simulink model "CAN_Tx"  (R2018b)
settings: Solver=FixedStepDiscrete  StartTime=0.0  StopTime=10.0  FixedStep=0.005  RelTol=1e-3
PostLoadFcn:
  | if any(exist('dsrtsu_mdlpostloadfcn', 'file') ~= 0), dsrtsu_mdlpostloadfcn('Execute', bdroot); end
values from neighbouring files (symbols this model uses):
  P_x165_On = 1.0    [CAN_Tx.sldd]
  P_x242_On = 1.0    [CAN_Tx.sldd]
  P_x246_On = 1.0    [CAN_Tx.sldd]
libraries: simulink x23, rtican x16
(part 2 of 4)

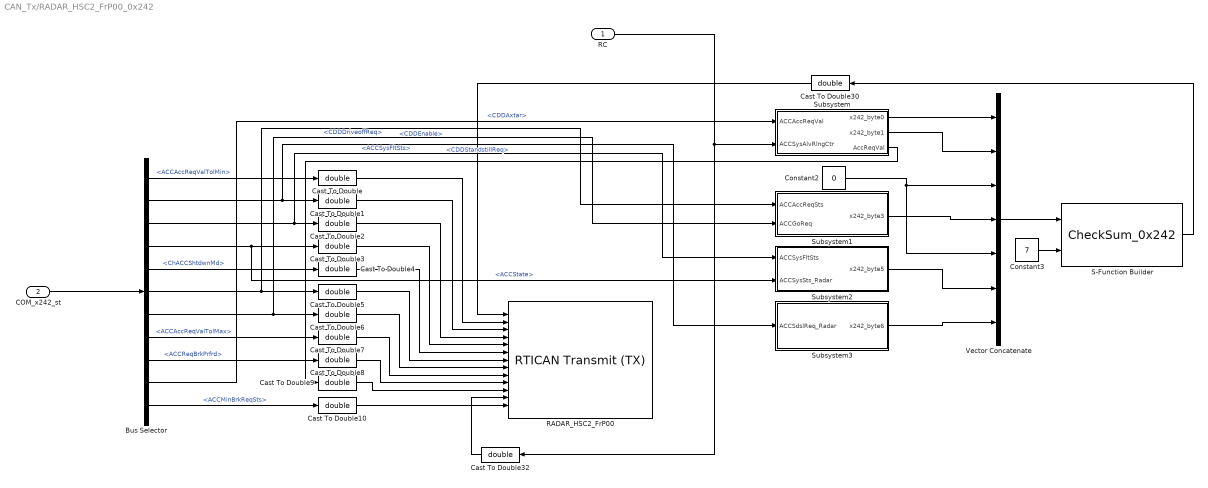
== system CAN_Tx/RADAR_HSC2_FrP00_0x242 ==
  RC : Inport
  COM_x242_st : Inport  Port=2
  Bus Selector : BusSelector  OutputSignals=ACCAccReqValTolMin,CDDStandstillReq,ACCSysFltSts,ACCState,ChACCShtdwnMd,CDDEnable,CDDDriveoffReq,ACCAccReqValTolMax,ACCReqBrkPrfrd,CDDAxtar,ACCMinBrkReqSts
  Cast To Double{,1..10,30,32} (13 alike) : DataTypeConversion  OutDataTypeStr=double
  Constant2 : Constant  Value=0  OutDataTypeStr=uint8
  Constant3 : Constant  Value=7  OutDataTypeStr=uint8
  RADAR_HSC2_FrP00 : rtican/RTICAN Transmit (TX)   Reserved1=[]  Reserved2=[]  Reserved3=[]  Reserved4=[]  SfcnMessage=[]  Msg_Struct=[]  BoardTypeNo=[]  BoardNo=[]  ChannelNo=[]  Parameters=[]  DialogFcn=[]  UnitName=[]  Revision=[]  UnitValues=[]  DSProperties=struct('RTI',struct('Version',uint32(5),'BlockType',struct('isSLSource',uint8(1),'isSLSink',uint8(1),'isHWSource',uint8(0),'isHWSink',uint8(0),'isSetup',uint8(0),'isInline',uint8(1),'isNonInline',uint8(0),'isInterrupt',uint8(0),'isChannelwise',uint8(0)),'IOBoardType','RTICAN','UnitType','MESSAGE','Identifier','TX','DialogType','MSVC','BlockSet','RTICAN','SlaveProcessor','CAN'))  RTIBlockInterface=struct('InputPortsWidth',int32([1 1 1 1 1 1 1 1 1 1 1 1 1]),'InputPortsActive',ones(1,13),'InputPortsName',{{'ACCSysChksm_SCSHSC2','ACCAccReqValTolMinHSC2','ACCSdslReq_RadarHSC2','ACCSysFltSts_SCSHSC2','ACCSysSts_RadarHSC2','ChACCShtdwnMdHSC2','ACCAccReqStsHSC2','ACCGoReqHSC2','ACCAccReqValTolMaxHSC2','ACCReqBrkPrfrdHSC2','ACCAccReqValHSC2','ACCSysAlvRlngCtr_SCSHSC2','ACCMinBrkReqStsHSC2'}},'InputPortsDataType',{{'SS_DOUBLE','SS_DOUBLE','SS_DOUBLE','SS_DOUBLE','SS_DOUBLE','SS_DOUBLE','SS_DOUBLE','SS_DOUBLE','SS_DOUBLE','SS_DOUBLE','SS_DOUBLE','SS_DOUBLE','SS_DOUBLE'}},'OutputPortsWidth',int32([1 1 1 1]),'OutputPortsActive',[1 1 1 1],'OutputPortsName',{{['TX status'],['TX time'],['TX delta time'],['TX delay time']}},'DialogFcn','rtican_message_interface_gui','BlockDisplay',{{'','center'}},'IconTransparency','on','InitLevel',3,'BlockName',struct('Token',{{'RADAR_HSC2_FrP00'}}),'SampleTime',{{-1}},'TriggerPort',{{'none'}},'EnablePort',{{'none'}})  RTIBlockParameters=struct('BoardTypeNo',{{1,'OFF',[]}},'BoardNo',{{1,'ON',[1 16]}},'ChannelNo',{{1,'ON',[1 2]}},'Parameters',{{struct('DataFileSupport',struct('DataFileSelectedMaster',1,'DataFileSelectedLocal',1,'DataFileName','c:\users\administrator.zx-201607042142\desktop\zone\2020_demo\ep21原车dbc\171114-lh1-ep21_ep2_fdr-_v07.dbc|','DataFileDate',['24-11月-2020 08:54:40'],'SelectedFile','..\..\dbc\ep21_dbc\171114-lh1-ep21_ep2_fdr-_v07_acc.dbc','InterfaceFcn','rtican_dbc_file_parser'),'Options',struct('StatusSelected',1,'TimeSelected',1,'DeltaTimeSelected',1,'DelayTimeSelected',1,'DelayTimeTXCommandSelected',0,'EncodeSetUnusedBitsToOne',0,'EnableMsgLoopback',0,'TriggerPort',struct('Selected',0,'TriggerType',0),'EnablePortSelected',0,'SignalOnPortnameSelected',1,'UserCoding',struct('Selected',0,'InterfaceFile','UserEncodingFile','FcnName','UserEncodeFcn','InportSelected',0,'InportWidth',1,'OutportSelected',0,'OutportWidth',1),'TerminationMsg',struct('Selected',0,'Byte0_7','0'),'InitialMsg',struct('Selected',0,'Byte0_7','0')),'Message',struct('MsgOnBlocknameSelected',1,'MsgName','RADAR_HSC2_FrP00','MsgIdFormat',0,'MsgId',578,'MsgLength',8,'NumSignals',13,'SampleTime',-1,'StartTime',struct('Selected',0,'Value',3),'AutoRepeatTime',struct('Selected',0,'Value',0.1),'Timeout',struct('Selected',0,'Value',0.1),'DelayTime',struct('Selected',0,'Value',0.1),'Signal',struct('SgnName',{'ACCSysChksm_SCSHSC2','ACCAccReqValTolMinHSC2','ACCSdslReq_RadarHSC2','ACCSysFltSts_SCSHSC2','ACCSysSts_RadarHSC2','ChACCShtdwnMdHSC2','ACCAccReqStsHSC2','ACCGoReqHSC2','ACCAccReqValTolMaxHSC2','ACCReqBrkPrfrdHSC2','ACCAccReqValHSC2','ACCSysAlvRlngCtr_SCSHSC2','ACCMinBrkReqStsHSC2'},'SgnStartBit',{0,8,15,16,19,22,36,38,40,47,48,59,63},'SgnLength',{8,7,1,3,3,2,2,1,7,1,11,4,1},'ByteLayout',{2,2,2,2,2,2,2,2,2,2,2,2,2},'Factor',{1,0.025,1,1,1,1,1,1,0.025,1,0.005,1,1},'Offset',{0,0,0,0,0,0,0,0,0,0,-7.22,0,0},'SgnComment',{'','','','','','',['Adaptive Cruise Control Acceleration Request Status'],['Adaptive Cruise Control Go Request'],'','','','',''},'SgnUnit',{'','','','','','','','','','','','',''},'Min',{0,0,0,0,0,0,0,0,0,0,-7.22,0,0},'Max',{255,3.175,1,7,7,3,3,1,3.175,1,3.015,15,1},'SgnType',{0,0,0,0,0,0,0,0,0,0,0,0,0},'SLDataType',{'SS_DOUBLE','SS_DOUBLE','SS_DOUBLE','SS_DOUBLE','SS_DOUBLE','SS_DOUBLE','SS_DOUBLE','SS_DOUBLE','SS_DOUBLE','SS_DOUBLE','SS_DOUBLE','SS_DOUBLE','SS_DOUBLE'},'DataType',{0,0,0,0,0,0,0,0,0,0,0,0,0},'ModeValue',{-1,-1,-1,-1,-1,-1,-1,-1,-1,-1,-1,-1,-1}),'MsgIdNumFormat',0,'MsgComment',{{''}}),'Version',1.2,'general',struct('isFromLib',0)),'OFF',[]}},'GroupId',{{struct('Group',{{'RTICAN'}},'No',1,'Behavior',{{'NAMECHANGE'}},'BlockType',{{'SINK'}},'NameChangeFlag',0),'OFF',[]}},'SFcnRTICANMessage',{{struct('MsgType','TX','SFcnPortType','Scalar','MsgName','RADAR_HSC2_FrP00','MsgIdFormat','STD','MsgId',578,'MsgLength',8,'NumSignals',13,'SampleTime',-1,'StartTime',struct('Selected','no','Value',3),'AutoRepeatTime',struct('Selected','no','Value',0.1),'Timeout',struct('Selected','no','Value',0.1),'Signal',struct('SgnName',{'ACCSysChksm_SCSHSC2','ACCAccReqValTolMinHSC2','ACCSdslReq_RadarHSC2','ACCSysFltSts_SCSHSC2','ACCSysSts_RadarHSC2','ChACCShtdwnMdHSC2','ACCAccReqStsHSC2','ACCGoReqHSC2','ACCAccReqValTolMaxHSC2','ACCReqBrkPrfrdHSC2','ACCAccReqValHSC2','ACCSysAlvRlngCtr_SCSHSC2','ACCMinBrkReqStsHSC2'},'SgnStartBit',{0,8,15,16,19,22,36,38,40,47,48,59,63},'SgnLength',{8,7,1,3,3,2,2,1,7,1,11,4,1},'ByteLayout',{['motorola back.'],['motorola back.'],['motorola back.'],['motorola back.'],['motorola back.'],['motorola back.'],['motorola back.'],['motorola back.'],['motorola back.'],['motorola back.'],['motorola back.'],['motorola back.'],['motorola back.']},'Factor',{1,0.025,1,1,1,1,1,1,0.025,1,0.005,1,1},'Offset',{0,0,0,0,0,0,0,0,0,0,-7.22,0,0},'SgnType',{'standard','standard','standard','standard','standard','standard','standard','standard','standard','standard','standard','standard','standard'},'SLDataType',{'SS_DOUBLE','SS_DOUBLE','SS_DOUBLE','SS_DOUBLE','SS_DOUBLE','SS_DOUBLE','SS_DOUBLE','SS_DOUBLE','SS_DOUBLE','SS_DOUBLE','SS_DOUBLE','SS_DOUBLE','SS_DOUBLE'},'DataType',{['unsigned int'],['unsigned int'],['unsigned int'],['unsigned int'],['unsigned int'],['unsigned int'],['unsigned int'],['unsigned int'],['unsigned int'],['unsigned int'],['unsigned int'],['unsigned int'],['unsigned int']},'ModeValue',{-1,-1,-1,-1,-1,-1,-1,-1,-1,-1,-1,-1,-1}),'StatusSelected','yes','TimeSelected','yes','DeltaTimeSelected','yes','DelayTimeSelected','yes','DelayTimeTXCommandSelected','no','EncodeSetUnusedBitsToOne','no','EnableMsgLoopback','no','TriggerPort',struct('Selected','no','TriggerType',0),'EnablePortSelected','no','UserCoding',struct('Selected','no','InterfaceFile','UserEncodingFile','FcnName','UserEncodeFcn','InportSelected','no','InportWidth',1,'OutportSelected','no','OutportWidth',1),'TerminationMsg',struct('Selected','no','Byte0','0x00','Byte1','0x00','Byte2','0x00','Byte3','0x00','Byte4','0x00','Byte5','0x00','Byte6','0x00','Byte7','0x00'),'InitialMsg',struct('Selected','no','Byte0','0x00','Byte1','0x00','Byte2','0x00','Byte3','0x00','Byte4','0x00','Byte5','0x00','Byte6','0x00','Byte7','0x00'),'BoardType','DS1','BoardNo',1,'ControllerNo',1),'OFF',[]}},'TLCFileName',{{'rtican_tx_message','OFF',[]}})  RTISFcnParameters=struct('SFcnRTICANMessage','struct','TLCFileName','char')  RTIBlockParaDefault=struct('BoardTypeNo',4302,'BoardNo',1,'ChannelNo',1,'Parameters',struct('DataFileSupport',struct('DataFileSelectedMaster',0,'DataFileSelectedLocal',0,'DataFileName','','DataFileDate','','SelectedFile',['<no file selected>']),'Options',struct('StatusSelected',1,'TimeSelected',1,'DeltaTimeSelected',1,'DelayTimeSelected',1,'DelayTimeTXCommandSelected',0,'EncodeSetUnusedBitsToOne',0,'EnableMsgLoopback',0,'TriggerPort',struct('Selected',0,'TriggerType','rising'),'EnablePortSelected',0,'SignalOnPortnameSelected',1,'UserCoding',struct('Selected',0,'InterfaceFile','UserEncodingFile','FcnName','UserEncodeFcn','InportSelected',0,'InportWidth',1,'OutportSelected',0,'OutportWidth',1),'TerminationMsg',struct('Selected',0,'Byte0_7','0'),'InitialMsg',struct('Selected',0,'Byte0_7','0')),'Message',struct('MsgOnBlocknameSelected',0,'MsgName',['TX Message'],'MsgIdFormat',0,'MsgId',100,'MsgLength',8,'NumSignals',1,'SampleTime',-1,'StartTime',struct('Selected',0,'Value',0),'AutoRepeatTime',struct('Selected',0,'Value',0.1),'Timeout',struct('Selected',0,'Value',0.1),'DelayTime',struct('Selected',0,'Value',0.1),'Signal',struct('SgnName',['TX signal'],'SgnStartBit',0,'SgnLength',8,'SgnType',0,'ModeValue',-1,'DataType',0,'SLDataType','SS_DOUBLE','ByteLayout',0,'Factor',1,'Offset',0,'Min',0,'Max',255,'SgnComment',{{}},'SgnUnit',''),'MsgIdNumFormat',0,'MsgComment',{{''}}),'Version',1.2,'general',struct('isFromLib',1)),'GroupId',struct('Group',{{'RTICAN'}},'No',1,'Behavior',{{'NAMECHANGE'}},'BlockType',{{'SINK'}},'NameChangeFlag',0),'SFcnRTICANMessage',struct('MsgType','TX','MsgName',['TX Message'],'MsgIdFormat','STD','MsgId',100,'MsgLength',2,'NumSignals',1,'SampleTime',-1,'StartTime',struct('Selected','no','Value',0),'AutoRepeatTime',struct('Selected','no','Value',0.1),'Timeout',struct('Selected','no','Value',0.1),'DelayTime',struct('Selected','no','Value',0.1),'Signal',struct('SgnName',['TX signal'],'SgnStartBit',0,'SgnLength',8,'SgnType','standard','ModeValue',-1,'DataType',['unsigned int'],'ByteLayout',['little endian'],'SLDataType','SS_DOUBLE','Factor',1,'Offset',0),'StatusSelected','yes','TimeSelected','yes','DeltaTimeSelected','yes','DelayTimeSelected','yes','EnablePortSelected','no','EnableMsgLoopback','no','DelayTimeTXCommandSelected','no','EncodeSetUnusedBitsToOne','no','UserCoding',struct('Selected','no','InterfaceFile','UserDecodingFile','FcnName','UserDecodeFcn','InportSelected','no','InportWidth',1,'OutportSelected','no','OutportWidth',1),'TerminationMsg',struct('Selected','no','Byte0','0x00','Byte1','0x00','Byte2','0x00','Byte3','0x00','Byte4','0x00','Byte5','0x00','Byte6','0x00','Byte7','0x00'),'InitialMsg',struct('Selected','no','Byte0','0x00','Byte1','0x00','Byte2','0x00','Byte3','0x00','Byte4','0x00','Byte5','0x00','Byte6','0x00','Byte7','0x00'),'TriggerPort',struct('Selected','no','TriggerType','rising'),'BoardType','DS4302','BoardNo',1,'ControllerNo',1,'SFcnPortType','Scalar'),'TLCFileName','rtican_tx_message')
      settings: AttributesFormatString=Group Id: RTICAN1\n  SourceProductName=dSPACE RTI CAN Blockset
  S-Function Builder : S-Function  InitFcn=try, set_param(gcb,'FunctionName','CheckSum_0x242'), end  FunctionName=CheckSum_0x242  SFunctionModules=CheckSum_0x242_wrapper  SFunctionDeploymentMode=off  EnableBusSupport=off  mask(S-Function Builder){}
      mask help: Simulink:masks:SFunctionBuilder_MD
      mask init:
      | val = [[.9  0.75 0.75 1 1 .9 .9 1]',[1 1 0.75 0.75 .9 .9 1 .9]'];try , sys = get_param(gcb,'SfunBuilderFcnName');if isempty(sys), sys = get_param(gcb,'FunctionName'); end,catch, sys = get_param(gcb,'FunctionName'); end
      settings: CopyFcn=set_param(gcbh,'LinkStatus','none')  PreSaveFcn=try, set_param(gcb,'FunctionName','CheckSum_0x242'), end  OpenFcn=sfunctionwizard(gcbh)
      mask Display: plot(val(:,1),val(:,2)),disp(sys), port_label('input',1,'data'), port_label('input',2,'length'), port_label('output',1,'u8_crc8')
  Subsystem : Subsystem
  Subsystem1 : Subsystem
  Subsystem2 : Subsystem
  Subsystem3 : Subsystem
  Vector Concatenate : Concatenate  NumInputs=7
  wires:
  Subsystem/1(x242_byte0) -> Vector Concatenate/1
  Cast To Double4/1 -> RADAR_HSC2_FrP00/6
  Subsystem/3(AccReqVal) -> Cast To Double9/1
  Bus Selector/5 -> Cast To Double4/1  "<ChACCShtdwnMd>"
  Bus Selector/6 -> Cast To Double5/1, Subsystem1/1(ACCAccReqSts)  "<CDDEnable>"
  Bus Selector/4 -> Cast To Double3/1, Subsystem2/2(ACCSysSts_Radar)  "<ACCState>"
  Bus Selector/7 -> Cast To Double6/1, Subsystem1/2(ACCGoReq)  "<CDDDriveoffReq>"
  Bus Selector/3 -> Cast To Double2/1, Subsystem2/1(ACCSysFltSts)  "<ACCSysFltSts>"
  Cast To Double32/1 -> RADAR_HSC2_FrP00/12
  S-Function Builder/1 -> Cast To Double30/1
  Bus Selector/10 -> Subsystem/1(ACCAccReqVal)  "<CDDAxtar>"
  Vector Concatenate/1 -> S-Function Builder/1
  Bus Selector/11 -> Cast To Double10/1  "<ACCMinBrkReqSts>"
  Cast To Double8/1 -> RADAR_HSC2_FrP00/10
  Cast To Double30/1 -> RADAR_HSC2_FrP00/1
  Cast To Double5/1 -> RADAR_HSC2_FrP00/7
  Bus Selector/1 -> Cast To Double/1  "<ACCAccReqValTolMin>"
  Cast To Double10/1 -> RADAR_HSC2_FrP00/13
  Cast To Double6/1 -> RADAR_HSC2_FrP00/8
  Subsystem3/1(x242_byte6) -> Vector Concatenate/7
  Constant3/1 -> S-Function Builder/2
  Bus Selector/8 -> Cast To Double7/1  "<ACCAccReqValTolMax>"
  Constant2/1 -> Vector Concatenate/5, Vector Concatenate/3
  Subsystem2/1(x242_byte5) -> Vector Concatenate/6
  Subsystem1/1(x242_byte3) -> Vector Concatenate/4
  Bus Selector/2 -> Cast To Double1/1, Subsystem3/1(ACCSdslReq_Radar)  "<CDDStandstillReq>"
  Cast To Double7/1 -> RADAR_HSC2_FrP00/9
  Cast To Double/1 -> RADAR_HSC2_FrP00/2
  Subsystem/2(x242_byte1) -> Vector Concatenate/2
  Cast To Double1/1 -> RADAR_HSC2_FrP00/3
  Cast To Double3/1 -> RADAR_HSC2_FrP00/5
  RC/1 -> Cast To Double32/1, Subsystem/2(ACCSysAlvRlngCtr)
  Cast To Double2/1 -> RADAR_HSC2_FrP00/4
  Bus Selector/9 -> Cast To Double8/1  "<ACCReqBrkPrfrd>"
  Cast To Double9/1 -> RADAR_HSC2_FrP00/11
  COM_x242_st/1 -> Bus Selector/1

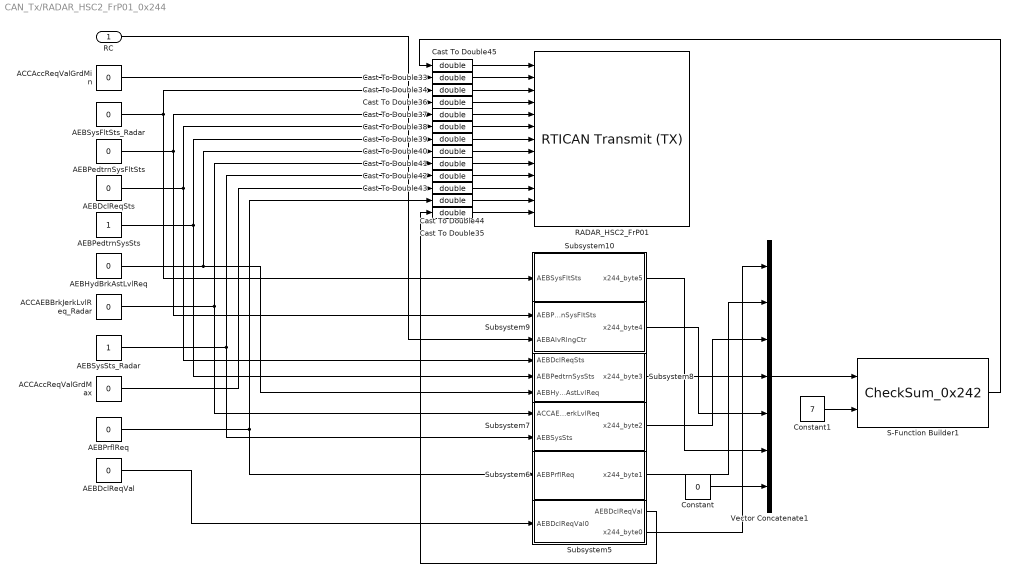
== system CAN_Tx/RADAR_HSC2_FrP01_0x244 ==
  RC : Inport
  ACCAEBBrkJerkLvlReq_Radar : Constant  Value=0  OutDataTypeStr=single
  ACCAccReqValGrdMax : Constant  Value=0  OutDataTypeStr=single
  ACCAccReqValGrdMin : Constant  Value=0  OutDataTypeStr=single
  AEBDclReqSts : Constant  Value=0  OutDataTypeStr=boolean
  AEBDclReqVal : Constant  Value=0  OutDataTypeStr=single
  AEBHydBrkAstLvlReq : Constant  Value=0  OutDataTypeStr=single
  AEBPedtrnSysFltSts : Constant  Value=0  OutDataTypeStr=single
  AEBPedtrnSysSts : Constant  OutDataTypeStr=single
  AEBPrflReq : Constant  Value=0  OutDataTypeStr=boolean
  AEBSysFltSts_Radar : Constant  Value=0  OutDataTypeStr=single
  AEBSysSts_Radar : Constant  OutDataTypeStr=single
  Cast To Double{33..45} (13 alike) : DataTypeConversion  OutDataTypeStr=double
  Constant : Constant  Value=0  OutDataTypeStr=uint8
  Constant1 : Constant  Value=7  OutDataTypeStr=uint8
  RADAR_HSC2_FrP01 : rtican/RTICAN Transmit (TX)   Reserved1=[]  Reserved2=[]  Reserved3=[]  Reserved4=[]  SfcnMessage=[]  Msg_Struct=[]  BoardTypeNo=[]  BoardNo=[]  ChannelNo=[]  Parameters=[]  DialogFcn=[]  UnitName=[]  Revision=[]  UnitValues=[]  DSProperties=struct('RTI',struct('Version',uint32(5),'BlockType',struct('isSLSource',uint8(1),'isSLSink',uint8(1),'isHWSource',uint8(0),'isHWSink',uint8(0),'isSetup',uint8(0),'isInline',uint8(1),'isNonInline',uint8(0),'isInterrupt',uint8(0),'isChannelwise',uint8(0)),'IOBoardType','RTICAN','UnitType','MESSAGE','Identifier','TX','DialogType','MSVC','BlockSet','RTICAN','SlaveProcessor','CAN'))  RTIBlockInterface=struct('InputPortsWidth',int32([1 1 1 1 1 1 1 1 1 1 1 1 1]),'InputPortsActive',ones(1,13),'InputPortsName',{{'AEBChksm_SCSHSC2','ACCAccReqValGrdMinHSC2','AEBSysFltSts_RadarHSC2','AEBAlvRlngCtr_SCSHSC2','AEBPedtrnSysFltStsHSC2','AEBDclReqStsHSC2','AEBPedtrnSysStsHSC2','AEBHydBrkAstLvlReqHSC2','ACCAEBBrkJerkLvlReq_RadarHSC2','AEBSysSts_RadarHSC2','ACCAccReqValGrdMaxHSC2','AEBPrflReqHSC2','AEBDclReqValHSC2'}},'InputPortsDataType',{{'SS_DOUBLE','SS_DOUBLE','SS_DOUBLE','SS_DOUBLE','SS_DOUBLE','SS_DOUBLE','SS_DOUBLE','SS_DOUBLE','SS_DOUBLE','SS_DOUBLE','SS_DOUBLE','SS_DOUBLE','SS_DOUBLE'}},'OutputPortsWidth',int32([1 1 1 1]),'OutputPortsActive',[1 1 1 1],'OutputPortsName',{{['TX status'],['TX time'],['TX delta time'],['TX delay time']}},'DialogFcn','rtican_message_interface_gui','BlockDisplay',{{'','center'}},'IconTransparency','on','InitLevel',3,'BlockName',struct('Token',{{'RADAR_HSC2_FrP01'}}),'SampleTime',{{-1}},'TriggerPort',{{'none'}},'EnablePort',{{'none'}})  RTIBlockParameters=struct('BoardTypeNo',{{1,'OFF',[]}},'BoardNo',{{1,'ON',[1 16]}},'ChannelNo',{{1,'ON',[1 2]}},'Parameters',{{struct('DataFileSupport',struct('DataFileSelectedMaster',1,'DataFileSelectedLocal',0,'DataFileName','c:\users\administrator.zx-201607042142\documents\matlab\dbc\ep21_dbc\171114-lh1-ep21_ep2_fdr-_v07.dbc|','DataFileDate',{{{['09-一月-2018 09:12:42']}}},'SelectedFile',['<no file selected>']),'Options',struct('StatusSelected',1,'TimeSelected',1,'DeltaTimeSelected',1,'DelayTimeSelected',1,'DelayTimeTXCommandSelected',0,'EncodeSetUnusedBitsToOne',0,'EnableMsgLoopback',0,'TriggerPort',struct('Selected',0,'TriggerType',0),'EnablePortSelected',0,'SignalOnPortnameSelected',1,'UserCoding',struct('Selected',0,'InterfaceFile','UserEncodingFile','FcnName','UserEncodeFcn','InportSelected',0,'InportWidth',1,'OutportSelected',0,'OutportWidth',1),'TerminationMsg',struct('Selected',0,'Byte0_7','0'),'InitialMsg',struct('Selected',0,'Byte0_7','0')),'Message',struct('MsgOnBlocknameSelected',1,'MsgName','RADAR_HSC2_FrP01','MsgIdFormat',0,'MsgId',580,'MsgLength',8,'NumSignals',13,'SampleTime',-1,'StartTime',struct('Selected',0,'Value',0),'AutoRepeatTime',struct('Selected',0,'Value',0.1),'Timeout',struct('Selected',0,'Value',0.1),'DelayTime',struct('Selected',0,'Value',0.1),'Signal',struct('SgnName',{'AEBChksm_SCSHSC2','ACCAccReqValGrdMinHSC2','AEBSysFltSts_RadarHSC2','AEBAlvRlngCtr_SCSHSC2','AEBPedtrnSysFltStsHSC2','AEBDclReqStsHSC2','AEBPedtrnSysStsHSC2','AEBHydBrkAstLvlReqHSC2','ACCAEBBrkJerkLvlReq_RadarHSC2','AEBSysSts_RadarHSC2','ACCAccReqValGrdMaxHSC2','AEBPrflReqHSC2','AEBDclReqValHSC2'},'SgnStartBit',{0,8,21,24,28,32,34,37,42,45,48,55,56},'SgnLength',{8,7,3,4,3,2,3,3,3,3,7,1,8},'SgnType',{0,0,0,0,0,0,0,0,0,0,0,0,0},'ModeValue',{-1,-1,-1,-1,-1,-1,-1,-1,-1,-1,-1,-1,-1},'DataType',{0,0,0,0,0,0,0,0,0,0,0,0,0},'ByteLayout',{2,2,2,2,2,2,2,2,2,2,2,2,2},'Factor',{1,0.1,1,1,1,1,1,1,1,1,0.1,1,0.1},'Offset',{0,-12.7,0,0,0,0,0,0,0,0,0,0,-12.7},'SgnComment',{{''},{['2017.05.23 updated:' char(10) 'ACCAEBBrkJerkReqValMin name changed to ACCAccReqValGrdMin']},{''},{''},{''},{['Autonomous Emergency Braking Deceleration Request Status']},{''},{''},{''},{''},{['2017.05.23:' char(10) 'ACCAEBBrkJerkReqValMax name changed to ACCAccReqValGrdMax']},{''},{['Autonomous Emergency Braking Deceleration Request Value']}},'SgnUnit',{'','','','','','','','','','','','','m/s^2'},'Min',{0,-12.7,0,0,0,0,0,0,0,0,0,0,-12.7},'Max',{255,3.7998e-7,7,15,7,3,7,7,7,7,12.7,1,12.8},'SLDataType',{'SS_DOUBLE','SS_DOUBLE','SS_DOUBLE','SS_DOUBLE','SS_DOUBLE','SS_DOUBLE','SS_DOUBLE','SS_DOUBLE','SS_DOUBLE','SS_DOUBLE','SS_DOUBLE','SS_DOUBLE','SS_DOUBLE'}),'MsgIdNumFormat',1,'MsgComment',{{''}}),'Version',1.2,'general',struct('isFromLib',0)),'OFF',[]}},'GroupId',{{struct('Group',{{'RTICAN'}},'No',1,'Behavior',{{'NAMECHANGE'}},'BlockType',{{'SINK'}},'NameChangeFlag',0),'OFF',[]}},'SFcnRTICANMessage',{{struct('MsgType','TX','SFcnPortType','Scalar','MsgName','RADAR_HSC2_FrP01','MsgIdFormat','STD','MsgId',580,'MsgLength',8,'NumSignals',13,'SampleTime',-1,'StartTime',struct('Selected','no','Value',0),'AutoRepeatTime',struct('Selected','no','Value',0.1),'Timeout',struct('Selected','no','Value',0.1),'Signal',struct('SgnName',{'AEBChksm_SCSHSC2','ACCAccReqValGrdMinHSC2','AEBSysFltSts_RadarHSC2','AEBAlvRlngCtr_SCSHSC2','AEBPedtrnSysFltStsHSC2','AEBDclReqStsHSC2','AEBPedtrnSysStsHSC2','AEBHydBrkAstLvlReqHSC2','ACCAEBBrkJerkLvlReq_RadarHSC2','AEBSysSts_RadarHSC2','ACCAccReqValGrdMaxHSC2','AEBPrflReqHSC2','AEBDclReqValHSC2'},'SgnStartBit',{0,8,21,24,28,32,34,37,42,45,48,55,56},'SgnLength',{8,7,3,4,3,2,3,3,3,3,7,1,8},'SgnType',{'standard','standard','standard','standard','standard','standard','standard','standard','standard','standard','standard','standard','standard'},'ModeValue',{-1,-1,-1,-1,-1,-1,-1,-1,-1,-1,-1,-1,-1},'DataType',{['unsigned int'],['unsigned int'],['unsigned int'],['unsigned int'],['unsigned int'],['unsigned int'],['unsigned int'],['unsigned int'],['unsigned int'],['unsigned int'],['unsigned int'],['unsigned int'],['unsigned int']},'ByteLayout',{['motorola back.'],['motorola back.'],['motorola back.'],['motorola back.'],['motorola back.'],['motorola back.'],['motorola back.'],['motorola back.'],['motorola back.'],['motorola back.'],['motorola back.'],['motorola back.'],['motorola back.']},'Factor',{1,0.1,1,1,1,1,1,1,1,1,0.1,1,0.1},'Offset',{0,-12.7,0,0,0,0,0,0,0,0,0,0,-12.7},'SLDataType',{'SS_DOUBLE','SS_DOUBLE','SS_DOUBLE','SS_DOUBLE','SS_DOUBLE','SS_DOUBLE','SS_DOUBLE','SS_DOUBLE','SS_DOUBLE','SS_DOUBLE','SS_DOUBLE','SS_DOUBLE','SS_DOUBLE'}),'StatusSelected','yes','TimeSelected','yes','DeltaTimeSelected','yes','DelayTimeSelected','yes','DelayTimeTXCommandSelected','no','EncodeSetUnusedBitsToOne','no','EnableMsgLoopback','no','TriggerPort',struct('Selected','no','TriggerType',0),'EnablePortSelected','no','UserCoding',struct('Selected','no','InterfaceFile','UserEncodingFile','FcnName','UserEncodeFcn','InportSelected','no','InportWidth',1,'OutportSelected','no','OutportWidth',1),'TerminationMsg',struct('Selected','no','Byte0','0x00','Byte1','0x00','Byte2','0x00','Byte3','0x00','Byte4','0x00','Byte5','0x00','Byte6','0x00','Byte7','0x00'),'InitialMsg',struct('Selected','no','Byte0','0x00','Byte1','0x00','Byte2','0x00','Byte3','0x00','Byte4','0x00','Byte5','0x00','Byte6','0x00','Byte7','0x00'),'BoardType','DS1','BoardNo',1,'ControllerNo',1),'OFF',[]}},'TLCFileName',{{'rtican_tx_message','OFF',[]}})  RTISFcnParameters=struct('SFcnRTICANMessage','struct','TLCFileName','char')  RTIBlockParaDefault=struct('BoardTypeNo',4302,'BoardNo',1,'ChannelNo',1,'Parameters',struct('DataFileSupport',struct('DataFileSelectedMaster',0,'DataFileSelectedLocal',0,'DataFileName','','DataFileDate','','SelectedFile',['<no file selected>']),'Options',struct('StatusSelected',1,'TimeSelected',1,'DeltaTimeSelected',1,'DelayTimeSelected',1,'DelayTimeTXCommandSelected',0,'EncodeSetUnusedBitsToOne',0,'EnableMsgLoopback',0,'TriggerPort',struct('Selected',0,'TriggerType','rising'),'EnablePortSelected',0,'SignalOnPortnameSelected',1,'UserCoding',struct('Selected',0,'InterfaceFile','UserEncodingFile','FcnName','UserEncodeFcn','InportSelected',0,'InportWidth',1,'OutportSelected',0,'OutportWidth',1),'TerminationMsg',struct('Selected',0,'Byte0_7','0'),'InitialMsg',struct('Selected',0,'Byte0_7','0')),'Message',struct('MsgOnBlocknameSelected',0,'MsgName',['TX Message'],'MsgIdFormat',0,'MsgId',100,'MsgLength',8,'NumSignals',1,'SampleTime',-1,'StartTime',struct('Selected',0,'Value',0),'AutoRepeatTime',struct('Selected',0,'Value',0.1),'Timeout',struct('Selected',0,'Value',0.1),'DelayTime',struct('Selected',0,'Value',0.1),'Signal',struct('SgnName',['TX signal'],'SgnStartBit',0,'SgnLength',8,'SgnType',0,'ModeValue',-1,'DataType',0,'SLDataType','SS_DOUBLE','ByteLayout',0,'Factor',1,'Offset',0,'Min',0,'Max',255,'SgnComment',{{}},'SgnUnit',''),'MsgIdNumFormat',0,'MsgComment',{{''}}),'Version',1.2,'general',struct('isFromLib',1)),'GroupId',struct('Group',{{'RTICAN'}},'No',1,'Behavior',{{'NAMECHANGE'}},'BlockType',{{'SINK'}},'NameChangeFlag',0),'SFcnRTICANMessage',struct('MsgType','TX','MsgName',['TX Message'],'MsgIdFormat','STD','MsgId',100,'MsgLength',2,'NumSignals',1,'SampleTime',-1,'StartTime',struct('Selected','no','Value',0),'AutoRepeatTime',struct('Selected','no','Value',0.1),'Timeout',struct('Selected','no','Value',0.1),'DelayTime',struct('Selected','no','Value',0.1),'Signal',struct('SgnName',['TX signal'],'SgnStartBit',0,'SgnLength',8,'SgnType','standard','ModeValue',-1,'DataType',['unsigned int'],'ByteLayout',['little endian'],'SLDataType','SS_DOUBLE','Factor',1,'Offset',0),'StatusSelected','yes','TimeSelected','yes','DeltaTimeSelected','yes','DelayTimeSelected','yes','EnablePortSelected','no','EnableMsgLoopback','no','DelayTimeTXCommandSelected','no','EncodeSetUnusedBitsToOne','no','UserCoding',struct('Selected','no','InterfaceFile','UserDecodingFile','FcnName','UserDecodeFcn','InportSelected','no','InportWidth',1,'OutportSelected','no','OutportWidth',1),'TerminationMsg',struct('Selected','no','Byte0','0x00','Byte1','0x00','Byte2','0x00','Byte3','0x00','Byte4','0x00','Byte5','0x00','Byte6','0x00','Byte7','0x00'),'InitialMsg',struct('Selected','no','Byte0','0x00','Byte1','0x00','Byte2','0x00','Byte3','0x00','Byte4','0x00','Byte5','0x00','Byte6','0x00','Byte7','0x00'),'TriggerPort',struct('Selected','no','TriggerType','rising'),'BoardType','DS4302','BoardNo',1,'ControllerNo',1,'SFcnPortType','Scalar'),'TLCFileName','rtican_tx_message')
      settings: AttributesFormatString=Group Id: RTICAN1\n  SourceProductName=dSPACE RTI CAN Blockset
  S-Function Builder1 : S-Function  InitFcn=try, set_param(gcb,'FunctionName','CheckSum_0x242'), end  FunctionName=CheckSum_0x242  SFunctionModules=CheckSum_0x242_wrapper  SFunctionDeploymentMode=off  EnableBusSupport=off  mask(S-Function Builder){}
      mask help: Simulink:masks:SFunctionBuilder_MD
      mask init: same as CAN_Tx/RADAR_HSC2_FrP00_0x242/S-Function Builder
      settings: CopyFcn=set_param(gcbh,'LinkStatus','none')  PreSaveFcn=try, set_param(gcb,'FunctionName','CheckSum_0x242'), end  OpenFcn=sfunctionwizard(gcbh)
      mask Display: plot(val(:,1),val(:,2)),disp(sys), port_label('input',1,'data'), port_label('input',2,'length'), port_label('output',1,'u8_crc8')
  Subsystem10 : Subsystem
  Subsystem5 : Subsystem
  Subsystem6 : Subsystem
  Subsystem7 : Subsystem
  Subsystem8 : Subsystem
  Subsystem9 : Subsystem
  Vector Concatenate1 : Concatenate  NumInputs=7
  wires:
  Constant1/1 -> S-Function Builder1/2
  Cast To Double33/1 -> RADAR_HSC2_FrP01/2
  Subsystem10/1(x244_byte5) -> Vector Concatenate1/6
  AEBPedtrnSysFltSts/1 -> Subsystem9/1(AEBPedtrnSysFltSts), Cast To Double37/1
  ACCAccReqValGrdMax/1 -> Cast To Double43/1
  AEBDclReqSts/1 -> Subsystem8/1(AEBDclReqSts), Cast To Double38/1
  Cast To Double40/1 -> RADAR_HSC2_FrP01/8
  AEBSysFltSts_Radar/1 -> Subsystem10/1(AEBSysFltSts), Cast To Double34/1
  AEBHydBrkAstLvlReq/1 -> Cast To Double40/1, Subsystem8/3(AEBHydBrkAstLvlReq)
  AEBPedtrnSysSts/1 -> Subsystem8/2(AEBPedtrnSysSts), Cast To Double39/1
  Cast To Double43/1 -> RADAR_HSC2_FrP01/11
  Subsystem8/1(x244_byte3) -> Vector Concatenate1/4
  Cast To Double38/1 -> RADAR_HSC2_FrP01/6
  Cast To Double34/1 -> RADAR_HSC2_FrP01/3
  S-Function Builder1/1 -> Cast To Double45/1
  Cast To Double35/1 -> RADAR_HSC2_FrP01/13
  Cast To Double41/1 -> RADAR_HSC2_FrP01/9
  Subsystem6/1(x244_byte1) -> Vector Concatenate1/2
  Cast To Double37/1 -> RADAR_HSC2_FrP01/5
  Cast To Double45/1 -> RADAR_HSC2_FrP01/1
  Constant/1 -> Vector Concatenate1/7
  AEBPrflReq/1 -> Cast To Double44/1, Subsystem6/1(AEBPrflReq)
  Cast To Double36/1 -> RADAR_HSC2_FrP01/4
  AEBDclReqVal/1 -> Subsystem5/1(AEBDclReqVal0)
  Vector Concatenate1/1 -> S-Function Builder1/1
  AEBSysSts_Radar/1 -> Cast To Double42/1, Subsystem7/2(AEBSysSts)
  Subsystem5/2(x244_byte0) -> Vector Concatenate1/1
  RC/1 -> Cast To Double36/1, Subsystem9/2(AEBAlvRlngCtr)
  Cast To Double42/1 -> RADAR_HSC2_FrP01/10
  Cast To Double39/1 -> RADAR_HSC2_FrP01/7
  Cast To Double44/1 -> RADAR_HSC2_FrP01/12
  Subsystem5/1(AEBDclReqVal) -> Cast To Double35/1
  ACCAccReqValGrdMin/1 -> Cast To Double33/1
  ACCAEBBrkJerkLvlReq_Radar/1 -> Subsystem7/1(ACCAEBBrkJerkLvlReq), Cast To Double41/1
  Subsystem7/1(x244_byte2) -> Vector Concatenate1/3
  Subsystem9/1(x244_byte4) -> Vector Concatenate1/5

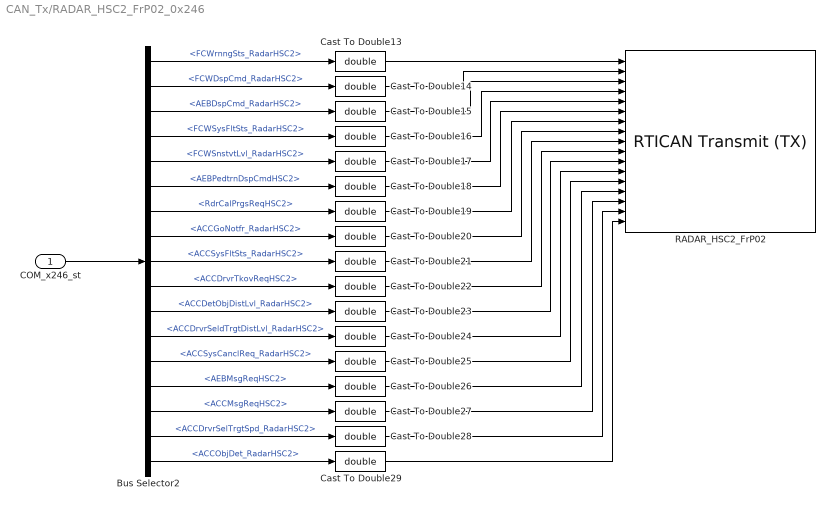
== system CAN_Tx/RADAR_HSC2_FrP02_0x246 ==
  COM_x246_st : Inport
  Bus Selector2 : BusSelector  OutputSignals=FCWrnngSts_RadarHSC2,FCWDspCmd_RadarHSC2,AEBDspCmd_RadarHSC2,FCWSysFltSts_RadarHSC2,FCWSnstvtLvl_RadarHSC2,AEBPedtrnDspCmdHSC2,RdrCalPrgsReqHSC2,ACCGoNotfr_RadarHSC2,ACCSysFltSts_RadarHSC2,ACCDrvrTkovReqHSC2,ACCDetObjDistLvl_RadarHSC2,ACCDrvrSeldTrgtDistLvl_RadarHSC2,ACCSysCanclReq_RadarHSC2,AEBMsgReqHSC2,ACCMsgReqHSC2,ACCDrvrSelTrgtSpd_RadarHSC2,ACCObjDet_RadarHSC2
  Cast To Double{13..29} (17 alike) : DataTypeConversion  OutDataTypeStr=double
  RADAR_HSC2_FrP02 : rtican/RTICAN Transmit (TX)   Reserved1=[]  Reserved2=[]  Reserved3=[]  Reserved4=[]  SfcnMessage=[]  Msg_Struct=[]  BoardTypeNo=[]  BoardNo=[]  ChannelNo=[]  Parameters=[]  DialogFcn=[]  UnitName=[]  Revision=[]  UnitValues=[]  DSProperties=struct('RTI',struct('Version',uint32(5),'BlockType',struct('isSLSource',uint8(1),'isSLSink',uint8(1),'isHWSource',uint8(0),'isHWSink',uint8(0),'isSetup',uint8(0),'isInline',uint8(1),'isNonInline',uint8(0),'isInterrupt',uint8(0),'isChannelwise',uint8(0)),'IOBoardType','RTICAN','UnitType','MESSAGE','Identifier','TX','DialogType','MSVC','BlockSet','RTICAN','SlaveProcessor','CAN'))  RTIBlockInterface=struct('InputPortsWidth',int32([1 1 1 1 1 1 1 1 1 1 1 1 1 1 1 1 1]),'InputPortsActive',ones(1,17),'InputPortsName',{{'FCWrnngSts_RadarHSC2','FCWDspCmd_RadarHSC2','AEBDspCmd_RadarHSC2','FCWSysFltSts_RadarHSC2','FCWSnstvtLvl_RadarHSC2','AEBPedtrnDspCmdHSC2','RdrCalPrgsReqHSC2','ACCGoNotfr_RadarHSC2','ACCSysFltSts_RadarHSC2','ACCDrvrTkovReqHSC2','ACCDetObjDistLvl_RadarHSC2','ACCDrvrSeldTrgtDistLvl_RadarHSC2','ACCSysCanclReq_RadarHSC2','AEBMsgReqHSC2','ACCMsgReqHSC2','ACCDrvrSelTrgtSpd_RadarHSC2','ACCObjDet_RadarHSC2'}},'InputPortsDataType',{{'SS_DOUBLE','SS_DOUBLE','SS_DOUBLE','SS_DOUBLE','SS_DOUBLE','SS_DOUBLE','SS_DOUBLE','SS_DOUBLE','SS_DOUBLE','SS_DOUBLE','SS_DOUBLE','SS_DOUBLE','SS_DOUBLE','SS_DOUBLE','SS_DOUBLE','SS_DOUBLE','SS_DOUBLE'}},'OutputPortsWidth',int32([1 1 1 1]),'OutputPortsActive',[1 1 1 1],'OutputPortsName',{{['TX status'],['TX time'],['TX delta time'],['TX delay time']}},'DialogFcn','rtican_message_interface_gui','BlockDisplay',{{'','center'}},'IconTransparency','on','InitLevel',3,'BlockName',struct('Token',{{'RADAR_HSC2_FrP02'}}),'SampleTime',{{-1}},'TriggerPort',{{'none'}},'EnablePort',{{'none'}})  RTIBlockParameters=struct('BoardTypeNo',{{1,'OFF',[]}},'BoardNo',{{1,'ON',[1 16]}},'ChannelNo',{{1,'ON',[1 2]}},'Parameters',{{struct('DataFileSupport',struct('DataFileSelectedMaster',1,'DataFileSelectedLocal',1,'DataFileName','c:\users\administrator.zx-201607042142\desktop\zone\2020_demo\ep21原车dbc\171114-lh1-ep21_ep2_fdr-_v07.dbc|','DataFileDate',['24-11月-2020 08:54:40'],'SelectedFile','..\..\dbc\ep21_dbc\171114-lh1-ep21_ep2_fdr-_v07_acc.dbc','InterfaceFcn','rtican_dbc_file_parser'),'Options',struct('StatusSelected',1,'TimeSelected',1,'DeltaTimeSelected',1,'DelayTimeSelected',1,'DelayTimeTXCommandSelected',0,'EncodeSetUnusedBitsToOne',0,'EnableMsgLoopback',0,'TriggerPort',struct('Selected',0,'TriggerType',0),'EnablePortSelected',0,'SignalOnPortnameSelected',1,'UserCoding',struct('Selected',0,'InterfaceFile','UserEncodingFile','FcnName','UserEncodeFcn','InportSelected',0,'InportWidth',1,'OutportSelected',0,'OutportWidth',1),'TerminationMsg',struct('Selected',0,'Byte0_7','0'),'InitialMsg',struct('Selected',0,'Byte0_7','0')),'Message',struct('MsgOnBlocknameSelected',1,'MsgName','RADAR_HSC2_FrP02','MsgIdFormat',0,'MsgId',582,'MsgLength',8,'NumSignals',17,'SampleTime',-1,'StartTime',struct('Selected',0,'Value',3),'AutoRepeatTime',struct('Selected',0,'Value',0.1),'Timeout',struct('Selected',0,'Value',0.1),'DelayTime',struct('Selected',0,'Value',0.1),'Signal',struct('SgnName',{'FCWrnngSts_RadarHSC2','FCWDspCmd_RadarHSC2','AEBDspCmd_RadarHSC2','FCWSysFltSts_RadarHSC2','FCWSnstvtLvl_RadarHSC2','AEBPedtrnDspCmdHSC2','RdrCalPrgsReqHSC2','ACCGoNotfr_RadarHSC2','ACCSysFltSts_RadarHSC2','ACCDrvrTkovReqHSC2','ACCDetObjDistLvl_RadarHSC2','ACCDrvrSeldTrgtDistLvl_RadarHSC2','ACCSysCanclReq_RadarHSC2','AEBMsgReqHSC2','ACCMsgReqHSC2','ACCDrvrSelTrgtSpd_RadarHSC2','ACCObjDet_RadarHSC2'},'SgnStartBit',{9,12,14,16,19,22,24,27,28,31,32,35,38,40,44,48,63},'SgnLength',{3,2,2,3,3,2,3,1,3,1,3,3,2,4,4,15,1},'ByteLayout',{2,2,2,2,2,2,2,2,2,2,2,2,2,2,2,2,2},'Factor',{1,1,1,1,1,1,1,1,1,1,1,1,1,1,1,2^-6,1},'Offset',{0,0,0,0,0,0,0,0,0,0,0,0,0,0,0,0,0},'SgnComment',{'','','','','','',['Radar Calibration Progress Request'],'','','','','','','','','',''},'SgnUnit',{'','','','','','','','','','','','','','','','',''},'Min',{0,0,0,0,0,0,0,0,0,0,0,0,0,0,0,0,0},'Max',{7,3,3,7,7,3,7,1,7,1,7,7,3,15,15,511.984,1},'SgnType',{0,0,0,0,0,0,0,0,0,0,0,0,0,0,0,0,0},'SLDataType',{'SS_DOUBLE','SS_DOUBLE','SS_DOUBLE','SS_DOUBLE','SS_DOUBLE','SS_DOUBLE','SS_DOUBLE','SS_DOUBLE','SS_DOUBLE','SS_DOUBLE','SS_DOUBLE','SS_DOUBLE','SS_DOUBLE','SS_DOUBLE','SS_DOUBLE','SS_DOUBLE','SS_DOUBLE'},'DataType',{0,0,0,0,0,0,0,0,0,0,0,0,0,0,0,0,0},'ModeValue',{-1,-1,-1,-1,-1,-1,-1,-1,-1,-1,-1,-1,-1,-1,-1,-1,-1}),'MsgIdNumFormat',0,'MsgComment',{{''}}),'Version',1.2,'general',struct('isFromLib',0)),'OFF',[]}},'GroupId',{{struct('Group',{{'RTICAN'}},'No',1,'Behavior',{{'NAMECHANGE'}},'BlockType',{{'SINK'}},'NameChangeFlag',0),'OFF',[]}},'SFcnRTICANMessage',{{struct('MsgType','TX','SFcnPortType','Scalar','MsgName','RADAR_HSC2_FrP02','MsgIdFormat','STD','MsgId',582,'MsgLength',8,'NumSignals',17,'SampleTime',-1,'StartTime',struct('Selected','no','Value',3),'AutoRepeatTime',struct('Selected','no','Value',0.1),'Timeout',struct('Selected','no','Value',0.1),'Signal',struct('SgnName',{'FCWrnngSts_RadarHSC2','FCWDspCmd_RadarHSC2','AEBDspCmd_RadarHSC2','FCWSysFltSts_RadarHSC2','FCWSnstvtLvl_RadarHSC2','AEBPedtrnDspCmdHSC2','RdrCalPrgsReqHSC2','ACCGoNotfr_RadarHSC2','ACCSysFltSts_RadarHSC2','ACCDrvrTkovReqHSC2','ACCDetObjDistLvl_RadarHSC2','ACCDrvrSeldTrgtDistLvl_RadarHSC2','ACCSysCanclReq_RadarHSC2','AEBMsgReqHSC2','ACCMsgReqHSC2','ACCDrvrSelTrgtSpd_RadarHSC2','ACCObjDet_RadarHSC2'},'SgnStartBit',{9,12,14,16,19,22,24,27,28,31,32,35,38,40,44,48,63},'SgnLength',{3,2,2,3,3,2,3,1,3,1,3,3,2,4,4,15,1},'ByteLayout',{['motorola back.'],['motorola back.'],['motorola back.'],['motorola back.'],['motorola back.'],['motorola back.'],['motorola back.'],['motorola back.'],['motorola back.'],['motorola back.'],['motorola back.'],['motorola back.'],['motorola back.'],['motorola back.'],['motorola back.'],['motorola back.'],['motorola back.']},'Factor',{1,1,1,1,1,1,1,1,1,1,1,1,1,1,1,2^-6,1},'Offset',{0,0,0,0,0,0,0,0,0,0,0,0,0,0,0,0,0},'SgnType',{'standard','standard','standard','standard','standard','standard','standard','standard','standard','standard','standard','standard','standard','standard','standard','standard','standard'},'SLDataType',{'SS_DOUBLE','SS_DOUBLE','SS_DOUBLE','SS_DOUBLE','SS_DOUBLE','SS_DOUBLE','SS_DOUBLE','SS_DOUBLE','SS_DOUBLE','SS_DOUBLE','SS_DOUBLE','SS_DOUBLE','SS_DOUBLE','SS_DOUBLE','SS_DOUBLE','SS_DOUBLE','SS_DOUBLE'},'DataType',{['unsigned int'],['unsigned int'],['unsigned int'],['unsigned int'],['unsigned int'],['unsigned int'],['unsigned int'],['unsigned int'],['unsigned int'],['unsigned int'],['unsigned int'],['unsigned int'],['unsigned int'],['unsigned int'],['unsigned int'],['unsigned int'],['unsigned int']},'ModeValue',{-1,-1,-1,-1,-1,-1,-1,-1,-1,-1,-1,-1,-1,-1,-1,-1,-1}),'StatusSelected','yes','TimeSelected','yes','DeltaTimeSelected','yes','DelayTimeSelected','yes','DelayTimeTXCommandSelected','no','EncodeSetUnusedBitsToOne','no','EnableMsgLoopback','no','TriggerPort',struct('Selected','no','TriggerType',0),'EnablePortSelected','no','UserCoding',struct('Selected','no','InterfaceFile','UserEncodingFile','FcnName','UserEncodeFcn','InportSelected','no','InportWidth',1,'OutportSelected','no','OutportWidth',1),'TerminationMsg',struct('Selected','no','Byte0','0x00','Byte1','0x00','Byte2','0x00','Byte3','0x00','Byte4','0x00','Byte5','0x00','Byte6','0x00','Byte7','0x00'),'InitialMsg',struct('Selected','no','Byte0','0x00','Byte1','0x00','Byte2','0x00','Byte3','0x00','Byte4','0x00','Byte5','0x00','Byte6','0x00','Byte7','0x00'),'BoardType','DS1','BoardNo',1,'ControllerNo',1),'OFF',[]}},'TLCFileName',{{'rtican_tx_message','OFF',[]}})  RTISFcnParameters=struct('SFcnRTICANMessage','struct','TLCFileName','char')  RTIBlockParaDefault=struct('BoardTypeNo',4302,'BoardNo',1,'ChannelNo',1,'Parameters',struct('DataFileSupport',struct('DataFileSelectedMaster',0,'DataFileSelectedLocal',0,'DataFileName','','DataFileDate','','SelectedFile',['<no file selected>']),'Options',struct('StatusSelected',1,'TimeSelected',1,'DeltaTimeSelected',1,'DelayTimeSelected',1,'DelayTimeTXCommandSelected',0,'EncodeSetUnusedBitsToOne',0,'EnableMsgLoopback',0,'TriggerPort',struct('Selected',0,'TriggerType','rising'),'EnablePortSelected',0,'SignalOnPortnameSelected',1,'UserCoding',struct('Selected',0,'InterfaceFile','UserEncodingFile','FcnName','UserEncodeFcn','InportSelected',0,'InportWidth',1,'OutportSelected',0,'OutportWidth',1),'TerminationMsg',struct('Selected',0,'Byte0_7','0'),'InitialMsg',struct('Selected',0,'Byte0_7','0')),'Message',struct('MsgOnBlocknameSelected',0,'MsgName',['TX Message'],'MsgIdFormat',0,'MsgId',100,'MsgLength',8,'NumSignals',1,'SampleTime',-1,'StartTime',struct('Selected',0,'Value',0),'AutoRepeatTime',struct('Selected',0,'Value',0.1),'Timeout',struct('Selected',0,'Value',0.1),'DelayTime',struct('Selected',0,'Value',0.1),'Signal',struct('SgnName',['TX signal'],'SgnStartBit',0,'SgnLength',8,'SgnType',0,'ModeValue',-1,'DataType',0,'SLDataType','SS_DOUBLE','ByteLayout',0,'Factor',1,'Offset',0,'Min',0,'Max',255,'SgnComment',{{}},'SgnUnit',''),'MsgIdNumFormat',0,'MsgComment',{{''}}),'Version',1.2,'general',struct('isFromLib',1)),'GroupId',struct('Group',{{'RTICAN'}},'No',1,'Behavior',{{'NAMECHANGE'}},'BlockType',{{'SINK'}},'NameChangeFlag',0),'SFcnRTICANMessage',struct('MsgType','TX','MsgName',['TX Message'],'MsgIdFormat','STD','MsgId',100,'MsgLength',2,'NumSignals',1,'SampleTime',-1,'StartTime',struct('Selected','no','Value',0),'AutoRepeatTime',struct('Selected','no','Value',0.1),'Timeout',struct('Selected','no','Value',0.1),'DelayTime',struct('Selected','no','Value',0.1),'Signal',struct('SgnName',['TX signal'],'SgnStartBit',0,'SgnLength',8,'SgnType','standard','ModeValue',-1,'DataType',['unsigned int'],'ByteLayout',['little endian'],'SLDataType','SS_DOUBLE','Factor',1,'Offset',0),'StatusSelected','yes','TimeSelected','yes','DeltaTimeSelected','yes','DelayTimeSelected','yes','EnablePortSelected','no','EnableMsgLoopback','no','DelayTimeTXCommandSelected','no','EncodeSetUnusedBitsToOne','no','UserCoding',struct('Selected','no','InterfaceFile','UserDecodingFile','FcnName','UserDecodeFcn','InportSelected','no','InportWidth',1,'OutportSelected','no','OutportWidth',1),'TerminationMsg',struct('Selected','no','Byte0','0x00','Byte1','0x00','Byte2','0x00','Byte3','0x00','Byte4','0x00','Byte5','0x00','Byte6','0x00','Byte7','0x00'),'InitialMsg',struct('Selected','no','Byte0','0x00','Byte1','0x00','Byte2','0x00','Byte3','0x00','Byte4','0x00','Byte5','0x00','Byte6','0x00','Byte7','0x00'),'TriggerPort',struct('Selected','no','TriggerType','rising'),'BoardType','DS4302','BoardNo',1,'ControllerNo',1,'SFcnPortType','Scalar'),'TLCFileName','rtican_tx_message')
      settings: AttributesFormatString=Group Id: RTICAN1\n  SourceProductName=dSPACE RTI CAN Blockset
  wires:
  Cast To Double21/1 -> RADAR_HSC2_FrP02/9
  Cast To Double20/1 -> RADAR_HSC2_FrP02/8
  Cast To Double23/1 -> RADAR_HSC2_FrP02/11
  Cast To Double28/1 -> RADAR_HSC2_FrP02/16
  Bus Selector2/7 -> Cast To Double19/1  "<RdrCalPrgsReqHSC2>"
  Cast To Double29/1 -> RADAR_HSC2_FrP02/17
  Bus Selector2/2 -> Cast To Double14/1  "<FCWDspCmd_RadarHSC2>"
  Cast To Double14/1 -> RADAR_HSC2_FrP02/2
  Bus Selector2/1 -> Cast To Double13/1  "<FCWrnngSts_RadarHSC2>"
  Cast To Double27/1 -> RADAR_HSC2_FrP02/15
  Cast To Double22/1 -> RADAR_HSC2_FrP02/10
  Cast To Double17/1 -> RADAR_HSC2_FrP02/5
  Cast To Double13/1 -> RADAR_HSC2_FrP02/1
  Bus Selector2/11 -> Cast To Double23/1  "<ACCDetObjDistLvl_RadarHSC2>"
  Bus Selector2/16 -> Cast To Double28/1  "<ACCDrvrSelTrgtSpd_RadarHSC2>"
  Cast To Double19/1 -> RADAR_HSC2_FrP02/7
  Cast To Double26/1 -> RADAR_HSC2_FrP02/14
  Bus Selector2/9 -> Cast To Double21/1  "<ACCSysFltSts_RadarHSC2>"
  Bus Selector2/5 -> Cast To Double17/1  "<FCWSnstvtLvl_RadarHSC2>"
  Cast To Double24/1 -> RADAR_HSC2_FrP02/12
  Bus Selector2/8 -> Cast To Double20/1  "<ACCGoNotfr_RadarHSC2>"
  Cast To Double18/1 -> RADAR_HSC2_FrP02/6
  Bus Selector2/6 -> Cast To Double18/1  "<AEBPedtrnDspCmdHSC2>"
  Bus Selector2/10 -> Cast To Double22/1  "<ACCDrvrTkovReqHSC2>"
  Bus Selector2/15 -> Cast To Double27/1  "<ACCMsgReqHSC2>"
  Bus Selector2/12 -> Cast To Double24/1  "<ACCDrvrSeldTrgtDistLvl_RadarHSC2>"
  Bus Selector2/3 -> Cast To Double15/1  "<AEBDspCmd_RadarHSC2>"
  Bus Selector2/14 -> Cast To Double26/1  "<AEBMsgReqHSC2>"
  COM_x246_st/1 -> Bus Selector2/1
  Cast To Double25/1 -> RADAR_HSC2_FrP02/13
  Bus Selector2/4 -> Cast To Double16/1  "<FCWSysFltSts_RadarHSC2>"
  Bus Selector2/17 -> Cast To Double29/1  "<ACCObjDet_RadarHSC2>"
  Bus Selector2/13 -> Cast To Double25/1  "<ACCSysCanclReq_RadarHSC2>"
  Cast To Double16/1 -> RADAR_HSC2_FrP02/4
  Cast To Double15/1 -> RADAR_HSC2_FrP02/3

== system CAN_Tx/RollingCounter ==
  Add2 : Sum
  Constant5 : Constant
  Constant6 : Constant  Value=-1
  Delay : Delay  DelayLength=1
  Switch : Switch  Criteria=u2 > Threshold  Threshold=14
  RC : Outport
  wires:
  Constant6/1 -> Switch/1
  Switch/1 -> Add2/2
  Delay/1 -> RC/1, Switch/3, Switch/2
  Add2/1 -> Delay/1
  Constant5/1 -> Add2/1
